simulink model "EV_EMR_2"  (R2024b)
settings: Solver=ode45  StartTime=SIM.t_min  StopTime=SIM.t_simul  FixedStep=1e-2  MaxStep=1e-3  RelTol=1e-3  EnableMultiTasking=on
InitFcn:
  | init_ev
values from neighbouring files (symbols this model uses):
  Ki_imot = 1    [init_ev.m]
  Kp_imot = 4    [init_ev.m]
undefined symbols (not defined in the file or in its folder): BATp, CHAp, CYCL, EMp, MTp, RDp
libraries: simulink x1
settings Model: Creator=Tony  LastModifiedBy=philippe.barrade
settings SolverCC: ZeroCrossAlgorithm=Non-adaptive  AlgebraicLoopSolver=TrustRegion
settings DataIOCC: SaveFormat=Array  SignalLoggingSaveFormat=ModelDataLogs  ReturnWorkspaceOutputs=off  SignalLoggingName=sigsOut
settings OptimizationCC: BooleanDataType=off  ExpressionDepthLimit=2147483647  LifeSpan=inf
settings DebuggingCC: SaveWithParameterizedLinksMsg=none  UnderspecifiedInitializationDetection=Classic  MergeDetectMultiDrivingBlocksExec=none  SignalResolutionControl=TryResolveAllWithWarning  MultiTaskDSMMsg=warning  MultiTaskCondExecSysMsg=none  FcnCallInpInsideContextMsg=warning  UnconnectedInputMsg=warning  UnconnectedOutputMsg=warning  UnconnectedLineMsg=warning  StateNameClashWarn=warning  SFUnexpectedBacktrackingDiag=warning  SFNoUnconditionalDefaultTransitionDiag=warning  ArithmeticOperatorsInVariantConditions=warning
settings HardwareCC: ProdBitPerPointer=32  ProdBitPerSizeT=32  ProdBitPerPtrDiffT=32  ProdLargestAtomicFloat=None  ProdIntDivRoundTo=Undefined  ProdEndianess=Unspecified  ProdWordSize=32  ProdHWDeviceType=32-bit Generic  TargetUnknown=on
settings ModelReferenceCC: EnableRefExpFcnMdlSchedulingChecks=on  PropagateSignalLabelsOutOfModel=off
settings SFSimCC: CustomCodeUndefinedFunction=UseInterfaceOnly
settings RTWCC: GPUComputeCapability=3.5
settings CodeAppCC: StateflowObjectComments=on
settings GRTTargetCC: TargetLangStandard=C89/C90 (ANSI)  CombineOutputUpdateFcns=off  GRTInterface=on
settings ConfigComp: CovMetricSettings=dw  CovSaveCumulativeToWorkspaceVar=on  CovSaveSingleToWorkspaceVar=on

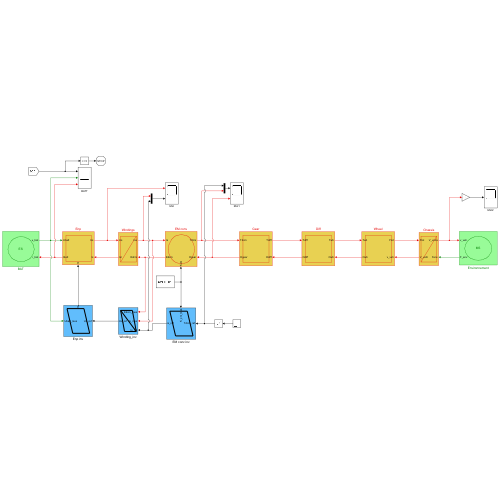
[thumbnail: Simulink's stored preview of the top-level diagram]
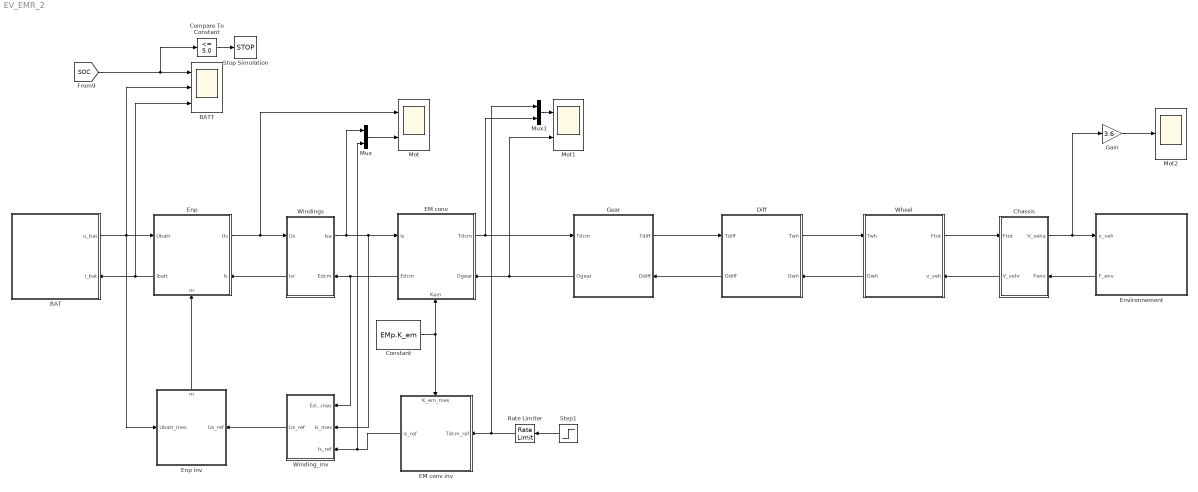
== system EV_EMR_2 ==
  BAT : Subsystem
      settings: PortSchema="{\"entries\":[{\"content\":{\"sides\":[{\"content\":{\"connectorIds\":[]},\"type\":\"ConnectorPlacement.EquallySpacedRectSide\",\"uuid\":\"f966fbbf-87fd-4eae-ac75-d366ea856ba9\"},{\"content\":{\"connectorIds\":[\"Out1\",\"In1\"],\"side\":\"RIGHT\"},\"type\":\"ConnectorPlacement.EquallySpacedRectSide\",\"uuid\":\"019a522f-a65b-4de4-928a-6ec503aa07e1\"},{\"content\":{\"connectorIds\":[],\"side\":\"TOP\"},\"type\":\"ConnectorPlacement.EquallySpacedRectSide\",\"uuid\":\"2e7350c2-17d6-436e-acd0-d7bc7ebcdc21\"}]},\"type\":\"ConnectorPlacement.EquallySpacedConnector\",\"uuid\":\"cf36ffa8-c853-4b91-8b40-e4ddcf06bdb1\"}],\"packageUris\":[\"http://schema.mathworks.com/mf0/Connector/R2020b\"],\"version\":\"1.0\"}"
      mask Display:
      | plot(0,0,100,100, 1.2*[50,57.68,60.77,63.08,64.97,66.58,68,69.26,70.4, 	71.42,72.36,78.28,80,78.28,72.36,71.42,70.4, 	69.26,68,66.58,64.97,63.08,60.77,57.68,50,42.32, 	39.23,36.92,35.03,33.42,32,30.74,29.6,28.58, 	27.64,21.72,20,21.72,27.64,28.58,29.6,30.74,32, 	33.42,35.03,36.92,39.23,42.32,50]-10, 1.2*[20,21,22,23,24,25,26,27,28,29,30,40,50,60,70,71,72, 	73,74,75,76,77,78,79,80,79,78,77,76,75,74,73,72, 	71,70,60,50,40,30,29,28,27,26,25,24,23,22,21,20]-10)
      | disp('ES')
  BATT : Scope  NumInputPorts=3
  Chassis : Subsystem  mask(CM){}
      settings: PortSchema="{\"entries\":[{\"content\":{\"sides\":[{\"content\":{\"connectorIds\":[\"In1\",\"Out2\"]},\"type\":\"ConnectorPlacement.EquallySpacedRectSide\",\"uuid\":\"620ffb90-6f06-474c-af56-4865758ad724\"},{\"content\":{\"connectorIds\":[\"Out1\",\"In2\"],\"side\":\"RIGHT\"},\"type\":\"ConnectorPlacement.EquallySpacedRectSide\",\"uuid\":\"7a4bba18-9bee-4c5d-b60c-6ae6fbfa3157\"},{\"content\":{\"connectorIds\":[],\"side\":\"TOP\"},\"type\":\"ConnectorPlacement.EquallySpacedRectSide\",\"uuid\":\"2f500b5d-e16a-4b09-8380-9fc4853d3c00\"}]},\"type\":\"ConnectorPlacement.EquallySpacedConnector\",\"uuid\":\"25a91873-aa5a-4f00-84d2-bf925e985f7d\"}],\"packageUris\":[\"http://schema.mathworks.com/mf0/Connector/R2020b\"],\"version\":\"1.0\"}"
      mask Display: plot(0,0,100,100,[10,10,90,90,10],[90,10,10,90,90], [10,90],[10,90])
  Compare To Constant : simulink/Logic and Bit Operations/Compare To Constant  relop=<=  const=5.0  OutDataTypeStr=boolean
  Constant : Constant  Value=EMp.K_em
  Diff : Subsystem  mask(Hacheur){}
      settings: PortSchema="{\"entries\":[{\"content\":{\"sides\":[{\"content\":{\"connectorIds\":[\"In1\",\"Out2\"]},\"type\":\"ConnectorPlacement.EquallySpacedRectSide\",\"uuid\":\"61fbc010-38ff-4a80-98f4-f5d8a9e77fd8\"},{\"content\":{\"connectorIds\":[\"Out1\",\"In2\"],\"side\":\"RIGHT\"},\"type\":\"ConnectorPlacement.EquallySpacedRectSide\",\"uuid\":\"7ae9e15d-ee0f-4ba6-b3b7-5dcbca441e0a\"},{\"content\":{\"connectorIds\":[],\"side\":\"TOP\"},\"type\":\"ConnectorPlacement.EquallySpacedRectSide\",\"uuid\":\"f4fbe656-3ef3-486e-b25e-f340040f3905\"},{\"content\":{\"connectorIds\":[],\"side\":\"BOTTOM\"},\"type\":\"ConnectorPlacement.EquallySpacedRectSide\",\"uuid\":\"e8cc994c-4958-42b4-b139-c82ce4c5ea4a\"}]},\"type\":\"ConnectorPlacement.EquallySpacedConnector\",\"uuid\":\"024d92c1-e2c4-4b69-9482-c403c9d240aa\"}],\"packageUris\":[\"http://schema.mathworks.com/mf0/Connector/R2020b\"],\"version\":\"1.0\"}"
      mask Display: plot(0,0,100,100,[10,10,90,90,10],[90,10,10,90,90])
  EM conv : Subsystem
      settings: PortSchema="{\"entries\":[{\"content\":{\"sides\":[{\"content\":{\"connectorIds\":[\"In1\",\"Out2\"]},\"type\":\"ConnectorPlacement.EquallySpacedRectSide\",\"uuid\":\"61fbc010-38ff-4a80-98f4-f5d8a9e77fd8\"},{\"content\":{\"connectorIds\":[\"Out1\",\"In3\"],\"side\":\"RIGHT\"},\"type\":\"ConnectorPlacement.EquallySpacedRectSide\",\"uuid\":\"7ae9e15d-ee0f-4ba6-b3b7-5dcbca441e0a\"},{\"content\":{\"connectorIds\":[],\"side\":\"TOP\"},\"type\":\"ConnectorPlacement.EquallySpacedRectSide\",\"uuid\":\"f4fbe656-3ef3-486e-b25e-f340040f3905\"},{\"content\":{\"connectorIds\":[\"In2\"],\"side\":\"BOTTOM\"},\"type\":\"ConnectorPlacement.EquallySpacedRectSide\",\"uuid\":\"742d13fb-c4a1-4c94-b7a0-3eefa6669287\"}]},\"type\":\"ConnectorPlacement.EquallySpacedConnector\",\"uuid\":\"024d92c1-e2c4-4b69-9482-c403c9d240aa\"}],\"packageUris\":[\"http://schema.mathworks.com/mf0/Connector/R2020b\"],\"version\":\"1.0\"}"
      mask Display: plot(0,0,100,100, 1.4*[50,57.68,60.77,63.08,64.97,66.58,68,69.26,70.4, 	71.42,72.36,78.28,80,78.28,72.36,71.42,70.4, 	69.26,68,66.58,64.97,63.08,60.77,57.68,50,42.32, 	39.23,36.92,35.03,33.42,32,30.74,29.6,28.58, 	27.64,21.72,20,21.72,27.64,28.58,29.6,30.74,32, 	33.42,35.03,36.92,39.23,42.32,50]-20, 1.4*[20,21,22,23,24,25,26,27,28,29,30,40,50,60,70,71,72, 	73,74,75,76,77,78,79,80,79,78,77,76,75,74,73,72, 	71,70,60,50,40,30,29,28,27,26,25,24,23,22,21,20]-20)
  EM conv inv : Subsystem
      settings: PortSchema="{\"entries\":[{\"content\":{\"sides\":[{\"content\":{\"connectorIds\":[\"In1\"]},\"type\":\"ConnectorPlacement.EquallySpacedRectSide\",\"uuid\":\"4d7f5df0-62dd-439c-ab7a-6b52334803c9\"},{\"content\":{\"connectorIds\":[\"Out1\"],\"side\":\"RIGHT\"},\"type\":\"ConnectorPlacement.EquallySpacedRectSide\",\"uuid\":\"e27848f4-b1e1-4693-91ac-f60d5fe9d3fd\"},{\"content\":{\"connectorIds\":[\"In2\"],\"side\":\"TOP\"},\"type\":\"ConnectorPlacement.EquallySpacedRectSide\",\"uuid\":\"3c2ec729-1d02-46dc-b19e-d40880938765\"}]},\"type\":\"ConnectorPlacement.EquallySpacedConnector\",\"uuid\":\"9d2baef6-6d4d-4c33-a220-4cfffab57276\"}],\"packageUris\":[\"http://schema.mathworks.com/mf0/Connector/R2020b\"],\"version\":\"1.0\"}"
      mask Display: plot(0,0,100,100,[10,30,90,70,10],[90,10,10,90,90])
  Enp : Subsystem  mask(Hacheur){}
      settings: PortSchema="{\"entries\":[{\"content\":{\"sides\":[{\"content\":{\"connectorIds\":[\"In1\",\"Out2\"]},\"type\":\"ConnectorPlacement.EquallySpacedRectSide\",\"uuid\":\"62d3361f-f49a-4a89-b7fa-c77fcee42868\"},{\"content\":{\"connectorIds\":[\"Out1\",\"In3\"],\"side\":\"RIGHT\"},\"type\":\"ConnectorPlacement.EquallySpacedRectSide\",\"uuid\":\"da99363c-611b-4582-b369-34120805217f\"},{\"content\":{\"side\":\"TOP\"},\"type\":\"ConnectorPlacement.EquallySpacedRectSide\",\"uuid\":\"7aa74fda-98a3-42bb-9007-2e39de70bf34\"},{\"content\":{\"connectorIds\":[\"In2\"],\"side\":\"BOTTOM\"},\"type\":\"ConnectorPlacement.EquallySpacedRectSide\",\"uuid\":\"47df5eac-c768-4899-b572-df26d6841fea\"}]},\"type\":\"ConnectorPlacement.EquallySpacedConnector\",\"uuid\":\"6baec6e9-7443-4760-93d1-cc70873952bd\"}],\"packageUris\":[\"http://schema.mathworks.com/mf0/Connector/R2020b\"],\"version\":\"1.0\"}"
      mask Display: plot(0,0,100,100,[10,10,90,90,10],[90,10,10,90,90])
  Enp inv : Subsystem
      settings: PortSchema="{\"entries\":[{\"content\":{\"sides\":[{\"content\":{\"connectorIds\":[\"In1\"]},\"type\":\"ConnectorPlacement.EquallySpacedRectSide\",\"uuid\":\"4d7f5df0-62dd-439c-ab7a-6b52334803c9\"},{\"content\":{\"connectorIds\":[\"In2\"],\"side\":\"RIGHT\"},\"type\":\"ConnectorPlacement.EquallySpacedRectSide\",\"uuid\":\"e27848f4-b1e1-4693-91ac-f60d5fe9d3fd\"},{\"content\":{\"connectorIds\":[\"Out1\"],\"side\":\"TOP\"},\"type\":\"ConnectorPlacement.EquallySpacedRectSide\",\"uuid\":\"3c2ec729-1d02-46dc-b19e-d40880938765\"}]},\"type\":\"ConnectorPlacement.EquallySpacedConnector\",\"uuid\":\"9d2baef6-6d4d-4c33-a220-4cfffab57276\"}],\"packageUris\":[\"http://schema.mathworks.com/mf0/Connector/R2020b\"],\"version\":\"1.0\"}"
      mask Display: plot(0,0,100,100,[10,30,90,70,10],[90,10,10,90,90])
  Environnement : Subsystem
      settings: PortSchema="{\"entries\":[{\"content\":{\"sides\":[{\"content\":{\"connectorIds\":[\"In1\",\"Out1\"]},\"type\":\"ConnectorPlacement.EquallySpacedRectSide\",\"uuid\":\"f966fbbf-87fd-4eae-ac75-d366ea856ba9\"},{\"content\":{\"connectorIds\":[],\"side\":\"RIGHT\"},\"type\":\"ConnectorPlacement.EquallySpacedRectSide\",\"uuid\":\"019a522f-a65b-4de4-928a-6ec503aa07e1\"},{\"content\":{\"connectorIds\":[],\"side\":\"TOP\"},\"type\":\"ConnectorPlacement.EquallySpacedRectSide\",\"uuid\":\"2e7350c2-17d6-436e-acd0-d7bc7ebcdc21\"}]},\"type\":\"ConnectorPlacement.EquallySpacedConnector\",\"uuid\":\"cf36ffa8-c853-4b91-8b40-e4ddcf06bdb1\"}],\"packageUris\":[\"http://schema.mathworks.com/mf0/Connector/R2020b\"],\"version\":\"1.0\"}"
      mask Display:
      | plot(0,0,100,100, 1.2*[50,57.68,60.77,63.08,64.97,66.58,68,69.26,70.4, 	71.42,72.36,78.28,80,78.28,72.36,71.42,70.4, 	69.26,68,66.58,64.97,63.08,60.77,57.68,50,42.32, 	39.23,36.92,35.03,33.42,32,30.74,29.6,28.58, 	27.64,21.72,20,21.72,27.64,28.58,29.6,30.74,32, 	33.42,35.03,36.92,39.23,42.32,50]-10, 1.2*[20,21,22,23,24,25,26,27,28,29,30,40,50,60,70,71,72, 	73,74,75,76,77,78,79,80,79,78,77,76,75,74,73,72, 	71,70,60,50,40,30,29,28,27,26,25,24,23,22,21,20]-10)
      | disp('MS')
  Gain : Gain  Gain=3.6
  Gear : Subsystem  mask(Hacheur){}
      settings: PortSchema="{\"entries\":[{\"content\":{\"sides\":[{\"content\":{\"connectorIds\":[\"In1\",\"Out2\"]},\"type\":\"ConnectorPlacement.EquallySpacedRectSide\",\"uuid\":\"61fbc010-38ff-4a80-98f4-f5d8a9e77fd8\"},{\"content\":{\"connectorIds\":[\"Out1\",\"In2\"],\"side\":\"RIGHT\"},\"type\":\"ConnectorPlacement.EquallySpacedRectSide\",\"uuid\":\"7ae9e15d-ee0f-4ba6-b3b7-5dcbca441e0a\"},{\"content\":{\"connectorIds\":[],\"side\":\"TOP\"},\"type\":\"ConnectorPlacement.EquallySpacedRectSide\",\"uuid\":\"f4fbe656-3ef3-486e-b25e-f340040f3905\"},{\"content\":{\"connectorIds\":[],\"side\":\"BOTTOM\"},\"type\":\"ConnectorPlacement.EquallySpacedRectSide\",\"uuid\":\"e8cc994c-4958-42b4-b139-c82ce4c5ea4a\"}]},\"type\":\"ConnectorPlacement.EquallySpacedConnector\",\"uuid\":\"024d92c1-e2c4-4b69-9482-c403c9d240aa\"}],\"packageUris\":[\"http://schema.mathworks.com/mf0/Connector/R2020b\"],\"version\":\"1.0\"}"
      mask Display: plot(0,0,100,100,[10,10,90,90,10],[90,10,10,90,90])
  Mot : Scope  NumInputPorts=2
  Mot1 : Scope  NumInputPorts=2
  Mot2 : Scope
  Mux : Mux  Inputs=2
  Mux1 : Mux  Inputs=2
  Rate Limiter : RateLimiter  RisingSlewLimit=EMp.T_max/0.5  FallingSlewLimit=-EMp.T_max/0.5  SampleTimeMode=inherited
  Step1 : Step  Time=100  Before=10.0  After=20.0  SampleTime=0
  Stop Simulation : Stop
  Wheel : Subsystem  mask(Hacheur){}
      settings: PortSchema="{\"entries\":[{\"content\":{\"sides\":[{\"content\":{\"connectorIds\":[\"In1\",\"Out2\"]},\"type\":\"ConnectorPlacement.EquallySpacedRectSide\",\"uuid\":\"61fbc010-38ff-4a80-98f4-f5d8a9e77fd8\"},{\"content\":{\"connectorIds\":[\"Out1\",\"In2\"],\"side\":\"RIGHT\"},\"type\":\"ConnectorPlacement.EquallySpacedRectSide\",\"uuid\":\"7ae9e15d-ee0f-4ba6-b3b7-5dcbca441e0a\"},{\"content\":{\"connectorIds\":[],\"side\":\"TOP\"},\"type\":\"ConnectorPlacement.EquallySpacedRectSide\",\"uuid\":\"f4fbe656-3ef3-486e-b25e-f340040f3905\"},{\"content\":{\"connectorIds\":[],\"side\":\"BOTTOM\"},\"type\":\"ConnectorPlacement.EquallySpacedRectSide\",\"uuid\":\"e8cc994c-4958-42b4-b139-c82ce4c5ea4a\"}]},\"type\":\"ConnectorPlacement.EquallySpacedConnector\",\"uuid\":\"024d92c1-e2c4-4b69-9482-c403c9d240aa\"}],\"packageUris\":[\"http://schema.mathworks.com/mf0/Connector/R2020b\"],\"version\":\"1.0\"}"
      mask Display: plot(0,0,100,100,[10,10,90,90,10],[90,10,10,90,90])
  Winding_inv : Subsystem  AncestorBlock=simulink/SMC/Asservissement Correcteur IP
      mask Display: plot(0,0,100,100, [10,30,90,70,10,90],[90,10,10,90,90,10])
  Windings : Subsystem  mask(CM){}
      settings: PortSchema="{\"entries\":[{\"content\":{\"sides\":[{\"content\":{\"connectorIds\":[\"In1\",\"Out2\"]},\"type\":\"ConnectorPlacement.EquallySpacedRectSide\",\"uuid\":\"620ffb90-6f06-474c-af56-4865758ad724\"},{\"content\":{\"connectorIds\":[\"Out1\",\"In2\"],\"side\":\"RIGHT\"},\"type\":\"ConnectorPlacement.EquallySpacedRectSide\",\"uuid\":\"7a4bba18-9bee-4c5d-b60c-6ae6fbfa3157\"},{\"content\":{\"connectorIds\":[],\"side\":\"TOP\"},\"type\":\"ConnectorPlacement.EquallySpacedRectSide\",\"uuid\":\"2f500b5d-e16a-4b09-8380-9fc4853d3c00\"}]},\"type\":\"ConnectorPlacement.EquallySpacedConnector\",\"uuid\":\"25a91873-aa5a-4f00-84d2-bf925e985f7d\"}],\"packageUris\":[\"http://schema.mathworks.com/mf0/Connector/R2020b\"],\"version\":\"1.0\"}"
      mask Display: plot(0,0,100,100,[10,10,90,90,10],[90,10,10,90,90], [10,90],[10,90])
  wires:
  BAT/1(u_bat) -> Enp inv/2(Ubatt_mes), Enp/1(Ubatt), BATT/2
  [SOC] -> Compare To Constant/1, BATT/1
  Compare To Constant/1 -> Stop Simulation/1
  Enp/2(Ibatt) -> BATT/3, BAT/1(i_bat)
  Enp inv/1(m) -> Enp/2(m)
  Enp/1(Us) -> Mot/1, Windings/1(Us)
  Windings/2(Isr) -> Enp/3(Is)
  Windings/1(Isa) -> Mux/1, Winding_inv/2(Is_mes), EM conv/1(Is)
  EM conv/2(Edcm) -> Winding_inv/1(Edcm_mes), Windings/2(Edcm)
  Constant/1 -> EM conv inv/2(K_em_mes), EM conv/2(Kem)
  Gear/2(Ogear) -> EM conv/3(Ogear), Mot1/2
  Winding_inv/1(Us_ref) -> Enp inv/1(Us_ref)
  Mux/1 -> Mot/2
  EM conv inv/1(is_ref) -> Mux/2, Winding_inv/3(Is_ref)
  Mux1/1 -> Mot1/1
  EM conv/1(Tdcm) -> Gear/1(Tdcm), Mux1/2
  Step1/1 -> Rate Limiter/1
  Rate Limiter/1 -> Mux1/1, EM conv inv/1(Tdcm_ref)
  Wheel/1(Ftot) -> Chassis/1(Ftot)
  Wheel/2(Owh) -> Diff/2(Owh)
  Chassis/2(V_vehr) -> Wheel/2(v_veh)
  Chassis/1(V_veha) -> Gain/1, Environnement/1(v_veh)
  Diff/2(Odiff) -> Gear/2(Odiff)
  Diff/1(Twh) -> Wheel/1(Twh)
  Gear/1(Tdiff) -> Diff/1(Tdiff)
  Environnement/1(F_env) -> Chassis/2(Fenv)
  Gain/1 -> Mot2/1

== system EV_EMR_2/BAT ==
  i_bat : Inport
  Adaptation : Subsystem  mask(CM){}
      settings: PortSchema="{\"entries\":[{\"content\":{\"sides\":[{\"content\":{\"connectorIds\":[\"In1\",\"Out2\"]},\"type\":\"ConnectorPlacement.EquallySpacedRectSide\",\"uuid\":\"43b53794-c784-4d35-8a91-f1490638489e\"},{\"content\":{\"connectorIds\":[\"Out1\",\"In2\"],\"side\":\"RIGHT\"},\"type\":\"ConnectorPlacement.EquallySpacedRectSide\",\"uuid\":\"00b1a1a6-7269-4083-abb9-f1208d9f3b4c\"},{\"content\":{\"connectorIds\":[],\"side\":\"TOP\"},\"type\":\"ConnectorPlacement.EquallySpacedRectSide\",\"uuid\":\"3919f87a-9a68-4334-b84e-5fe8c9917a96\"}]},\"type\":\"ConnectorPlacement.EquallySpacedConnector\",\"uuid\":\"9597a696-d499-48cc-bc44-63d792d74754\"}],\"packageUris\":[\"http://schema.mathworks.com/mf0/Connector/R2020b\"],\"version\":\"1.0\"}"
      mask Display: plot(0,0,100,100, [10,10,90,90,10],[90,10,10,90,90], [90,10,90],[10,50,90])
  Battery  cell resistance : Subsystem  mask(Hacheur){}
      settings: PortSchema="{\"entries\":[{\"content\":{\"sides\":[{\"content\":{\"connectorIds\":[\"In1\",\"Out2\"]},\"type\":\"ConnectorPlacement.EquallySpacedRectSide\",\"uuid\":\"43b53794-c784-4d35-8a91-f1490638489e\"},{\"content\":{\"connectorIds\":[\"Out1\",\"In2\"],\"side\":\"RIGHT\"},\"type\":\"ConnectorPlacement.EquallySpacedRectSide\",\"uuid\":\"00b1a1a6-7269-4083-abb9-f1208d9f3b4c\"},{\"content\":{\"connectorIds\":[],\"side\":\"TOP\"},\"type\":\"ConnectorPlacement.EquallySpacedRectSide\",\"uuid\":\"3919f87a-9a68-4334-b84e-5fe8c9917a96\"}]},\"type\":\"ConnectorPlacement.EquallySpacedConnector\",\"uuid\":\"9597a696-d499-48cc-bc44-63d792d74754\"}],\"packageUris\":[\"http://schema.mathworks.com/mf0/Connector/R2020b\"],\"version\":\"1.0\"}"
      mask Display: plot(0,0,100,100,[10,10,90,90,10],[90,10,10,90,90])
  OCV Source : Subsystem
      settings: PortSchema="{\"entries\":[{\"content\":{\"sides\":[{\"content\":{\"connectorIds\":[]},\"type\":\"ConnectorPlacement.EquallySpacedRectSide\",\"uuid\":\"87b7c904-bcc3-4a98-87e1-6b58a76e8897\"},{\"content\":{\"connectorIds\":[\"Out1\",\"In1\"],\"side\":\"RIGHT\"},\"type\":\"ConnectorPlacement.EquallySpacedRectSide\",\"uuid\":\"67c0e4e9-ec6a-4f26-b099-e0fb0eaa0b35\"},{\"content\":{\"connectorIds\":[],\"side\":\"TOP\"},\"type\":\"ConnectorPlacement.EquallySpacedRectSide\",\"uuid\":\"8fb5181e-f6b7-4828-b0d6-b00809980f9d\"}]},\"type\":\"ConnectorPlacement.EquallySpacedConnector\",\"uuid\":\"ac4387ff-8ed1-4b4c-b503-b7c8237b5a9a\"}],\"packageUris\":[\"http://schema.mathworks.com/mf0/Connector/R2020b\"],\"version\":\"1.0\"}"
      mask Display:
      | plot(0,0,100,100, 1.2*[50,57.68,60.77,63.08,64.97,66.58,68,69.26,70.4, 	71.42,72.36,78.28,80,78.28,72.36,71.42,70.4, 	69.26,68,66.58,64.97,63.08,60.77,57.68,50,42.32, 	39.23,36.92,35.03,33.42,32,30.74,29.6,28.58, 	27.64,21.72,20,21.72,27.64,28.58,29.6,30.74,32, 	33.42,35.03,36.92,39.23,42.32,50]-10, 1.2*[20,21,22,23,24,25,26,27,28,29,30,40,50,60,70,71,72, 	73,74,75,76,77,78,79,80,79,78,77,76,75,74,73,72, 	71,70,60,50,40,30,29,28,27,26,25,24,23,22,21,20]-10)
      | disp('MS')
  u_bat : Outport  InitialOutput=0
  wires:
  Adaptation/1(u_bat) -> u_bat/1
  i_bat/1 -> Adaptation/2(I_bat)
  Adaptation/2(i_cell) -> Battery  cell resistance/2(icell)
  Battery  cell resistance/1(u_cell) -> Adaptation/1(u_cell)
  OCV Source/1(OCV) -> Battery  cell resistance/1(OCV)
  Battery  cell resistance/2(I_cell) -> OCV Source/1("I_cell ")

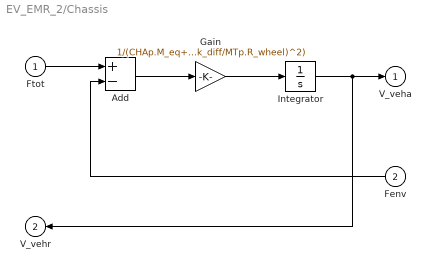
== system EV_EMR_2/Chassis ==
  Ftot : Inport
  Fenv : Inport  Port=2
  Add : Sum  Inputs=+-
  Gain : Gain  Gain=1/(CHAp.M_eq+EMp.J*(MTp.k_gear*MTp.k_diff/MTp.R_wheel)^2)
  Integrator : Integrator
  V_veha : Outport  InitialOutput=0
  V_vehr : Outport  Port=2  InitialOutput=0
  wires:
  Ftot/1 -> Add/1
  Add/1 -> Gain/1
  Gain/1 -> Integrator/1
  Integrator/1 -> V_veha/1, V_vehr/1
  Fenv/1 -> Add/2

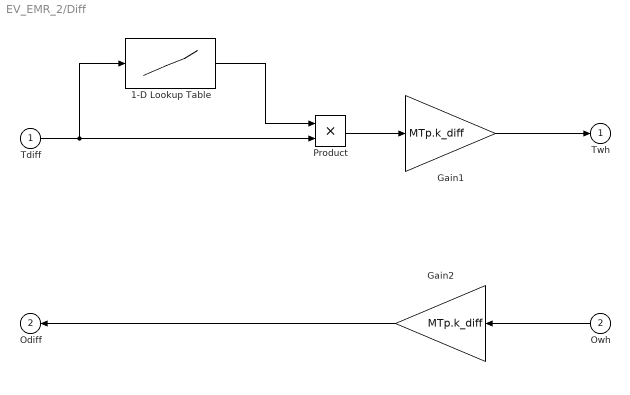
== system EV_EMR_2/Diff ==
  Tdiff : Inport
  Owh : Inport  Port=2
  1-D Lookup Table : Lookup_n-D  NumberOfTableDimensions=1  BreakpointsForDimension1=[-500 -200 -10 0 10 200 500]  Table=[1/MTp.diff_eff 1/MTp.diff_eff 1/MTp.diff_eff 0 MTp.diff_eff MTp.diff_eff MTp.diff_eff]  InternalRulePriority=Speed  RndMeth=Simplest
  Gain1 : Gain  Gain=MTp.k_diff
  Gain2 : Gain  Gain=MTp.k_diff
  Product : Product
  Twh : Outport  InitialOutput=0
  Odiff : Outport  Port=2  InitialOutput=0
  wires:
  Gain1/1 -> Twh/1
  Tdiff/1 -> Product/2, 1-D Lookup Table/1
  Gain2/1 -> Odiff/1
  Owh/1 -> Gain2/1
  Product/1 -> Gain1/1
  1-D Lookup Table/1 -> Product/1

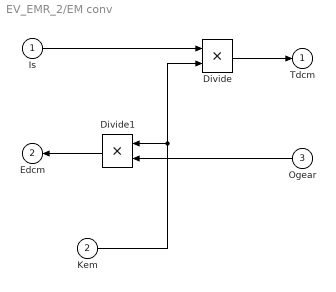
== system EV_EMR_2/EM conv ==
  Is : Inport
  Kem : Inport  Port=2
  Ogear : Inport  Port=3
  Divide : Product  Inputs=**
  Divide1 : Product  Inputs=**
  Tdcm : Outport  InitialOutput=0
  Edcm : Outport  Port=2  InitialOutput=0
  wires:
  Is/1 -> Divide/1
  Divide/1 -> Tdcm/1
  Divide1/1 -> Edcm/1
  Ogear/1 -> Divide1/2
  Kem/1 -> Divide1/1, Divide/2

== system EV_EMR_2/EM conv inv ==
  Tdcm_ref : Inport
  K_em_mes : Inport  Port=2
  Product : Product  Inputs=/*
  Saturation : Saturate  UpperLimit=Inf  LowerLimit=0.1
  is_ref : Outport  InitialOutput=0
  wires:
  K_em_mes/1 -> Saturation/1
  Tdcm_ref/1 -> Product/2
  Product/1 -> is_ref/1
  Saturation/1 -> Product/1

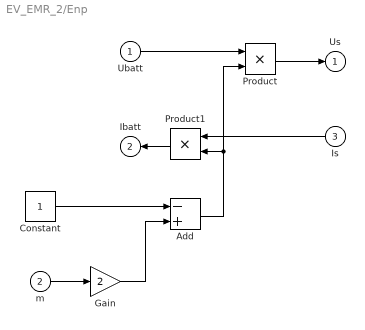
== system EV_EMR_2/Enp ==
  Ubatt : Inport
  m : Inport  Port=2
  Is : Inport  Port=3
  Add : Sum  Inputs=-+
  Constant : Constant
  Gain : Gain  Gain=2
  Product : Product
  Product1 : Product
  Us : Outport  InitialOutput=0
  Ibatt : Outport  Port=2  InitialOutput=0
  wires:
  m/1 -> Gain/1
  Constant/1 -> Add/1
  Gain/1 -> Add/2
  Product/1 -> Us/1
  Ubatt/1 -> Product/1
  Add/1 -> Product1/2, Product/2
  Product1/1 -> Ibatt/1
  Is/1 -> Product1/1

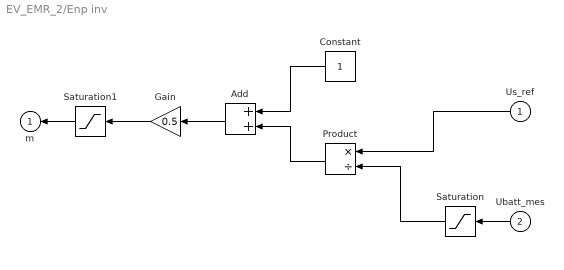
== system EV_EMR_2/Enp inv ==
  Us_ref : Inport
  Ubatt_mes : Inport  Port=2
  Add : Sum
  Constant : Constant
  Gain : Gain  Gain=0.5
  Product : Product  Inputs=*/
  Saturation : Saturate  UpperLimit=Inf  LowerLimit=10
  Saturation1 : Saturate  UpperLimit=1  LowerLimit=0
  m : Outport  InitialOutput=0
  wires:
  Ubatt_mes/1 -> Saturation/1
  Us_ref/1 -> Product/1
  Saturation/1 -> Product/2
  Constant/1 -> Add/1
  Product/1 -> Add/2
  Add/1 -> Gain/1
  Gain/1 -> Saturation1/1
  Saturation1/1 -> m/1

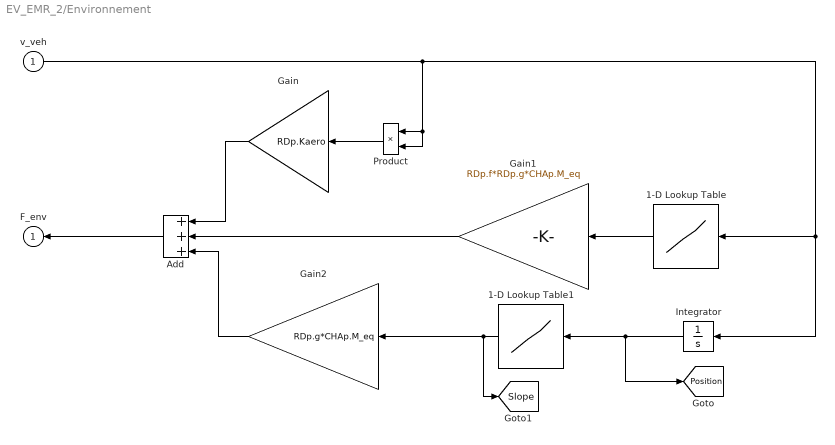
== system EV_EMR_2/Environnement ==
  v_veh : Inport
  1-D Lookup Table : Lookup_n-D  NumberOfTableDimensions=1  BreakpointsForDimension1=[-100 -1 0 1 100]  Table=[-1 -1 0 1 1]  InternalRulePriority=Speed  RndMeth=Simplest
  1-D Lookup Table1 : Lookup_n-D  NumberOfTableDimensions=1  BreakpointsForDimension1=CYCL.position  Table=CYCL.slope  InternalRulePriority=Speed  RndMeth=Simplest
  Add : Sum  Inputs=+++
  Gain : Gain  Gain=RDp.Kaero  SaturateOnIntegerOverflow=on  OutDataTypeStr=Inherit: Same as input  ParamDataTypeStr=Inherit: Same as input
  Gain1 : Gain  Gain=RDp.f*RDp.g*CHAp.M_eq  SaturateOnIntegerOverflow=on  OutDataTypeStr=Inherit: Same as input  ParamDataTypeStr=Inherit: Same as input
  Gain2 : Gain  Gain=RDp.g*CHAp.M_eq  SaturateOnIntegerOverflow=on  OutDataTypeStr=Inherit: Same as input  ParamDataTypeStr=Inherit: Same as input
  Integrator : Integrator
  Product : Product  InputSameDT=on  SaturateOnIntegerOverflow=on  OutDataTypeStr=Inherit: Same as first input
  F_env : Outport  InitialOutput=0
  tag scope: Position=global, Slope=global
  wires:
  Product/1 -> Gain/1
  Add/1 -> F_env/1
  v_veh/1 -> Product/1, Product/2, Integrator/1, 1-D Lookup Table/1
  Gain/1 -> Add/1
  Gain1/1 -> Add/2
  1-D Lookup Table/1 -> Gain1/1
  Integrator/1 -> [Position], 1-D Lookup Table1/1
  1-D Lookup Table1/1 -> Gain2/1, [Slope]
  Gain2/1 -> Add/3

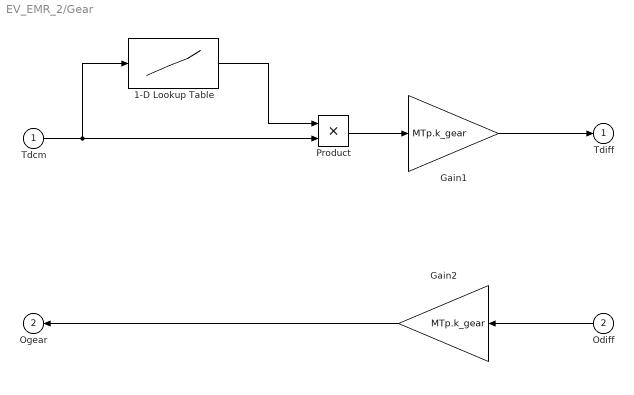
== system EV_EMR_2/Gear ==
  Tdcm : Inport
  Odiff : Inport  Port=2
  1-D Lookup Table : Lookup_n-D  NumberOfTableDimensions=1  BreakpointsForDimension1=[-500 -200 -10 0 10 200 500]  Table=[1/MTp.Gear_eff 1/MTp.Gear_eff 1/MTp.Gear_eff 0 MTp.Gear_eff MTp.Gear_eff MTp.Gear_eff]  InternalRulePriority=Speed  RndMeth=Simplest
  Gain1 : Gain  Gain=MTp.k_gear
  Gain2 : Gain  Gain=MTp.k_gear
  Product : Product
  Tdiff : Outport  InitialOutput=0
  Ogear : Outport  Port=2  InitialOutput=0
  wires:
  Gain1/1 -> Tdiff/1
  Tdcm/1 -> Product/2, 1-D Lookup Table/1
  Gain2/1 -> Ogear/1
  Odiff/1 -> Gain2/1
  Product/1 -> Gain1/1
  1-D Lookup Table/1 -> Product/1

== system EV_EMR_2/Wheel ==
  Twh : Inport
  v_veh : Inport  Port=2
  Gain1 : Gain  Gain=1/MTp.R_wheel
  Gain2 : Gain  Gain=1/MTp.R_wheel
  Ftot : Outport  InitialOutput=0
  Owh : Outport  Port=2  InitialOutput=0
  wires:
  Gain1/1 -> Ftot/1
  Gain2/1 -> Owh/1
  v_veh/1 -> Gain2/1
  Twh/1 -> Gain1/1

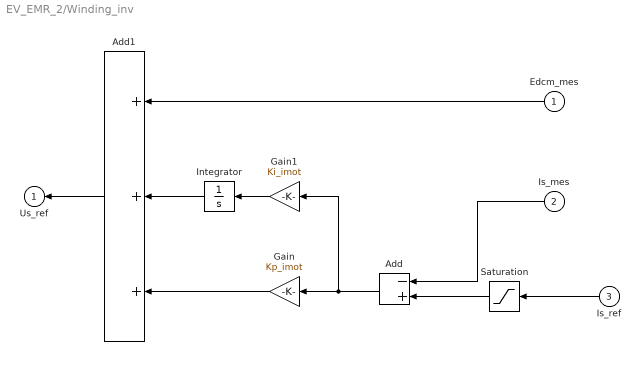
== system EV_EMR_2/Winding_inv ==
  Edcm_mes : Inport
  Is_mes : Inport  Port=2
  Is_ref : Inport  Port=3
  Add : Sum  Inputs=-+
  Add1 : Sum  Inputs=+++
  Gain : Gain  Gain=Kp_imot
  Gain1 : Gain  Gain=Ki_imot
  Integrator : Integrator
  Saturation : Saturate  UpperLimit=EMp.I_arm_max  LowerLimit=-EMp.I_arm_max
  Us_ref : Outport  InitialOutput=0
  wires:
  Is_ref/1 -> Saturation/1
  Is_mes/1 -> Add/1
  Add1/1 -> Us_ref/1
  Add/1 -> Gain1/1, Gain/1
  Gain1/1 -> Integrator/1
  Gain/1 -> Add1/3
  Integrator/1 -> Add1/2
  Edcm_mes/1 -> Add1/1
  Saturation/1 -> Add/2

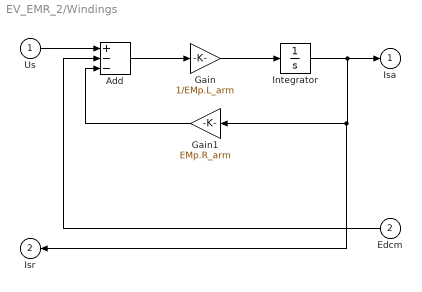
== system EV_EMR_2/Windings ==
  Us : Inport
  Edcm : Inport  Port=2
  Add : Sum  Inputs=+--
  Gain : Gain  Gain=1/EMp.L_arm
  Gain1 : Gain  Gain=EMp.R_arm
  Integrator : Integrator
  Isa : Outport  InitialOutput=0
  Isr : Outport  Port=2  InitialOutput=0
  wires:
  Us/1 -> Add/1
  Add/1 -> Gain/1
  Gain/1 -> Integrator/1
  Integrator/1 -> Isa/1, Isr/1, Gain1/1
  Gain1/1 -> Add/3
  Edcm/1 -> Add/2

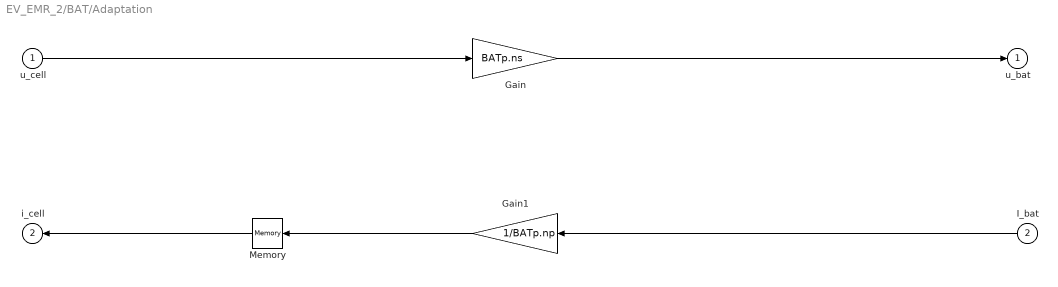
== system EV_EMR_2/BAT/Adaptation ==
  u_cell : Inport
  I_bat : Inport  Port=2
  Gain : Gain  Gain=BATp.ns
  Gain1 : Gain  Gain=1/BATp.np
  Memory : Memory
  u_bat : Outport  InitialOutput=0
  i_cell : Outport  Port=2  InitialOutput=0
  wires:
  Gain/1 -> u_bat/1
  I_bat/1 -> Gain1/1
  u_cell/1 -> Gain/1
  Gain1/1 -> Memory/1
  Memory/1 -> i_cell/1

== system EV_EMR_2/BAT/Battery  cell resistance ==
  OCV : Inport
  icell : Inport  Port=2
  Gain : Gain  Gain=BATp.Rcell
  Subtract : Sum  Inputs=+-
  u_cell : Outport  InitialOutput=0
  I_cell : Outport  Port=2  InitialOutput=0
  wires:
  Subtract/1 -> u_cell/1
  icell/1 -> I_cell/1, Gain/1
  Gain/1 -> Subtract/2
  OCV/1 -> Subtract/1

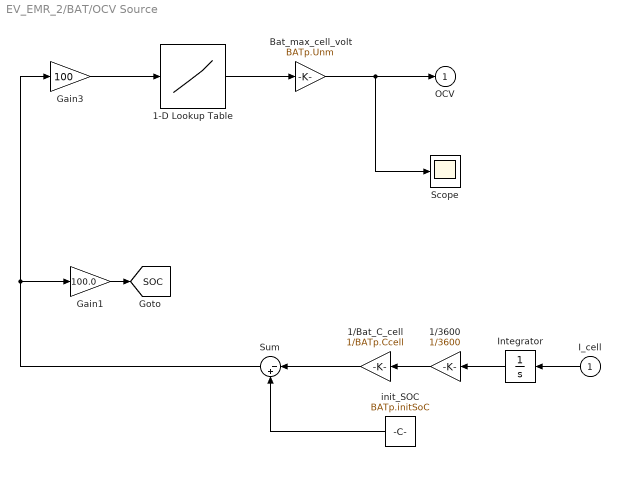
== system EV_EMR_2/BAT/OCV Source ==
  "I_cell " : Inport
  1-D Lookup Table : Lookup_n-D  NumberOfTableDimensions=1  BreakpointsForDimension1=BATp.SoC  Table=BATp.OCV  InternalRulePriority=Speed  RndMeth=Simplest
  1/3600 : Gain  Gain=1/3600
  1/Bat_C_cell : Gain  Gain=1/BATp.Ccell
  Bat_max_cell_volt : Gain  Gain=BATp.Unm
  Gain1 : Gain  Gain=100.0
  Gain3 : Gain  Gain=100
  Integrator : Integrator
  Scope : Scope
  Sum : Sum  Inputs=|-+
  init_SOC : Constant  Value=BATp.initSoC
  OCV : Outport  InitialOutput=0
  tag scope: SOC=global
  wires:
  Sum/1 -> Gain1/1, Gain3/1
  1-D Lookup Table/1 -> Bat_max_cell_volt/1
  Gain3/1 -> 1-D Lookup Table/1
  Integrator/1 -> 1/3600/1
  init_SOC/1 -> Sum/2
  1/Bat_C_cell/1 -> Sum/1
  "I_cell "/1 -> Integrator/1
  1/3600/1 -> 1/Bat_C_cell/1
  Bat_max_cell_volt/1 -> Scope/1, OCV/1
  Gain1/1 -> [SOC]
